simulink model "StateTransition_MRCC"  (R2016a)
settings: Solver=FixedStepDiscrete  StartTime=0.0  StopTime=320  FixedStep=0.1  RelTol=1e-3
settings Model: SimulationMode=accelerator  NumberOfSteps=5  Creator=id  LastModifiedBy=id
settings SolverCC: AutoInsertRateTranBlk=on
settings DataIOCC: LimitDataPoints=on
settings DebuggingCC: AllowSymbolicDim=off
settings GRTTargetCC: GeneratePreprocessorConditionals=Use local settings

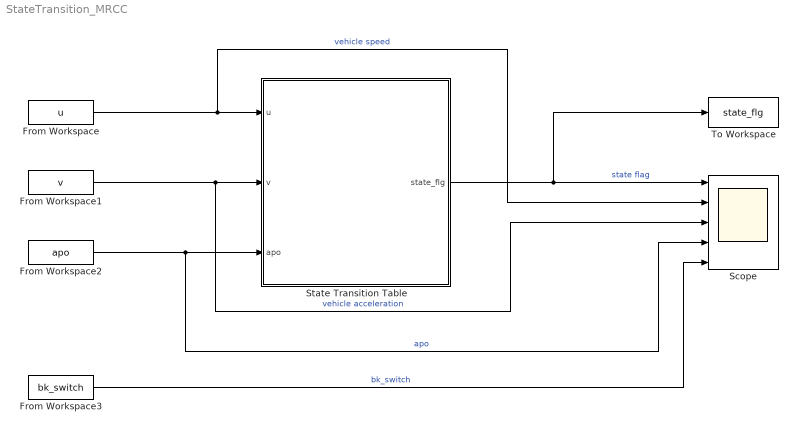
== system StateTransition_MRCC ==
  From Workspace : FromWorkspace  VariableName=u  SampleTime=0
  From Workspace1 : FromWorkspace  VariableName=v  SampleTime=0
  From Workspace2 : FromWorkspace  VariableName=apo  SampleTime=0
  From Workspace3 : FromWorkspace  VariableName=bk_switch  SampleTime=0
  Scope : Scope  NumInputPorts=5
  State Transition Table : State Transition Table  TreatAsAtomicUnit=on
  To Workspace : ToWorkspace  VariableName=state_flg  SaveFormat=Timeseries  SampleTime=-1
  wires:
  From Workspace/1 -> State Transition Table/1(u), Scope/2  "vehicle speed"
  From Workspace1/1 -> Scope/3, State Transition Table/2(v)  "vehicle acceleration"
  State Transition Table/1(state_flg) -> To Workspace/1, Scope/1  "state flag"
  From Workspace2/1 -> Scope/4, State Transition Table/3(apo)  "apo"
  From Workspace3/1 -> Scope/5  "bk_switch"

== stateflow chart StateTransition_MRCC/State Transition Table ==
  state Accel
    entry: state_flg = 1;
  state Decel1
    entry: state_flg = 2;
  state Coast
    entry: state_flg = 3;
  state Cruise
    entry: state_flg = 4;
  state Idle
    entry: state_flg = 0;
  (default) -> Accel
  Accel -> (junction 69) [order 1] : [(u < 0.5 && v>=0.02) || (v>0.1) ] %accel condition
  (junction 69) -> Accel
  (junction 253) -> Accel
  (junction 750) -> (junction 253)
  Accel -> (junction 440) [order 5] : [(u <= 0.5 && v<0.02 && v>-0.02) || (v<0.02) ] %idle condition
  (junction 440) -> (junction 489)
  Accel -> (junction 766) [order 3] : [ ((u > 0.5 && v<0.02 && v>-0.02)) && apo==0  ] %coast condition
  (junction 766) -> (junction 757)
  Accel -> (junction 775) [order 4] : [ ((u > 0.5 && v<0.02 && v>-0.02)) && apo>0  ] %cruise condition
  (junction 775) -> (junction 778)
  Accel -> Decel1 [order 2] : [(u > 0.5 && v<=-0.02) || (v<-0.02) ] %decel condition
  Decel1 -> Accel [order 2] : [(u < 0.5 && v>=0.02) || (v>0.1) ] %accel condition
  Decel1 -> (junction 75) [order 1] : [(u > 0.5 && v<=-0.02) || (v<-0.02) ] %decel condition
  (junction 75) -> Decel1
  (junction 261) -> Decel1
  (junction 788) -> (junction 261)
  Decel1 -> (junction 489) [order 5] : [(u <= 0.5 && v<0.02 && v>-0.02) || (v<0.02) ] %idle condition
  (junction 489) -> (junction 754)
  Decel1 -> (junction 778) [order 4] : [ ((u > 0.5 && v<0.02 && v>-0.02)) && apo>0  ] %cruise condition
  (junction 778) -> (junction 773)
  Decel1 -> Coast [order 3] : [ ((u > 0.5 && v<0.02 && v>-0.02)) && apo==0  ] %coast condition
  Coast -> Decel1 [order 3] : [(u > 0.5 && v<=-0.02) || (v<-0.02) ] %decel condition
  Coast -> (junction 747) [order 1] : [ ((u > 0.5 && v<0.02 && v>-0.02)) && apo==0  ] %coast condition
  (junction 747) -> Coast
  Coast -> (junction 750) [order 2] : [(u < 0.5 && v>=0.02) || (v>0.1) ] %accel condition
  (junction 785) -> (junction 750)
  Coast -> (junction 754) [order 5] : [(u <= 0.5 && v<0.02 && v>-0.02) || (v<0.02) ] %idle condition
  (junction 754) -> (junction 226)
  (junction 757) -> Coast
  (junction 782) -> (junction 757)
  Coast -> Cruise [order 4] : [ ((u > 0.5 && v<0.02 && v>-0.02)) && apo>0  ] %cruise condition
  Cruise -> Coast [order 4] : [ ((u > 0.5 && v<0.02 && v>-0.02)) && apo==0  ] %coast condition
  Cruise -> (junction 668) [order 1] : [ ((u > 0.5 && v<0.02 && v>-0.02)) && apo>0  ] %cruise condition
  (junction 668) -> Cruise
  Cruise -> (junction 785) [order 2] : [(u < 0.5 && v>=0.02) || (v>0.1) ] %accel condition
  (junction 268) -> (junction 785)
  Cruise -> (junction 788) [order 3] : [(u > 0.5 && v<=-0.02) || (v<-0.02) ] %decel condition
  (junction 773) -> Cruise
  (junction 271) -> (junction 788)
  Cruise -> Idle [order 5] : [(u <= 0.5 && v<0.02 && v>-0.02) || (v<0.02) ] %idle condition
  Idle -> Cruise [order 5] : [ ((u > 0.5 && v<0.02 && v>-0.02)) && apo>0  ] %cruise condition
  Idle -> (junction 87) [order 1] : [(u <= 0.5 && v<0.02 && v>-0.02) || (v<0.02) ] %idle condition
  (junction 87) -> Idle
  Idle -> (junction 268) [order 2] : [(u < 0.5 && v>=0.02) || (v>0.1) ] %accel condition
  Idle -> (junction 271) [order 3] : [(u > 0.5 && v<=-0.02) || (v<-0.02) ] %decel condition
  (junction 226) -> Idle
  Idle -> (junction 782) [order 4] : [ ((u > 0.5 && v<0.02 && v>-0.02)) && apo==0  ] %coast condition
  data: u input; v input; state_flg output; apo input
